simulink model "PurePursuit"  (R2020b)
settings: Solver=VariableStepAuto  StartTime=0  StopTime=10  RelTol=1e-3
undefined symbols (not defined in the file or in its folder): map, parking_space, start_pos
libraries: Solver_SF x1
settings Model: Creator=ASCL-321  LastModifiedBy=ASCL-321

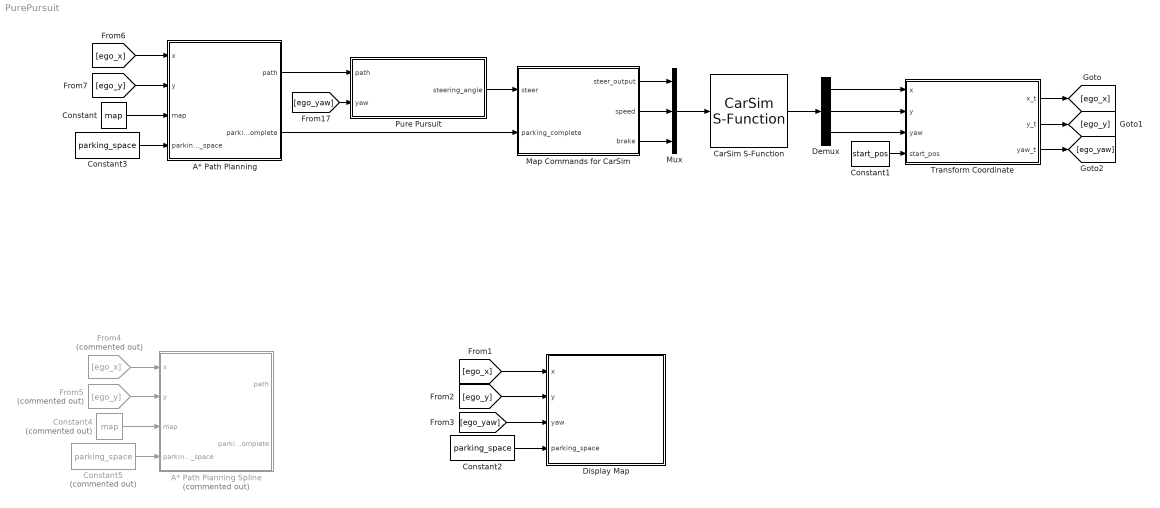
== system PurePursuit ==
  A* Path Planning : MATLAB Function  TreatAsAtomicUnit=on  SystemSampleTime=0.1
  A* Path Planning Spline : MATLAB Function  Commented=on  TreatAsAtomicUnit=on  SystemSampleTime=0.1
  CarSim S-Function : Solver_SF/CarSim S-Function  Priority=1  SIMFILE=simfile.sim  Run_RTs=off  vs_state_ind=Run  StopMode_ind=Vehicle Model
  Constant : Constant  Value=map
  Constant1 : Constant  Value=start_pos
  Constant2 : Constant  Value=parking_space
  Constant3 : Constant  Value=parking_space
  Constant4 : Constant  Commented=on  Value=map
  Constant5 : Constant  Commented=on  Value=parking_space
  Demux : Demux  Outputs=3
  Display Map : MATLAB Function  TreatAsAtomicUnit=on  SystemSampleTime=0.1
  From4 : From  Commented=on  GotoTag=ego_x
  From5 : From  Commented=on  GotoTag=ego_y
  Map Commands for CarSim : MATLAB Function  TreatAsAtomicUnit=on  SystemSampleTime=0.1
  Mux : Mux  Inputs=3
  Pure Pursuit : MATLAB Function  TreatAsAtomicUnit=on  SystemSampleTime=0.1
  Transform Coordinate : MATLAB Function  TreatAsAtomicUnit=on  SystemSampleTime=0.1
  wires:
  Map Commands for CarSim/1(steer_output) -> Mux/1
  Map Commands for CarSim/2(speed) -> Mux/2
  Mux/1 -> CarSim S-Function/1
  A* Path Planning/1(path) -> Pure Pursuit/1(path)
  CarSim S-Function/1 -> Demux/1
  Demux/1 -> Transform Coordinate/1(x)
  Demux/2 -> Transform Coordinate/2(y)
  [ego_yaw] -> Pure Pursuit/2(yaw)
  [ego_x] -> Display Map/1(x)
  [ego_y] -> Display Map/2(y)
  Demux/3 -> Transform Coordinate/3(yaw)
  [ego_yaw] -> Display Map/3(yaw)
  Transform Coordinate/3(yaw_t) -> [ego_yaw]
  Transform Coordinate/1(x_t) -> [ego_x]
  Transform Coordinate/2(y_t) -> [ego_y]
  Map Commands for CarSim/3(brake) -> Mux/3
  A* Path Planning/2(parking_complete) -> Map Commands for CarSim/2(parking_complete)
  Constant1/1 -> Transform Coordinate/4(start_pos)
  Constant2/1 -> Display Map/4(parking_space)
  Pure Pursuit/1(steering_angle) -> Map Commands for CarSim/1(steer)
  Constant/1 -> A* Path Planning/3(map)
  [ego_x] -> A* Path Planning/1(x)
  Constant3/1 -> A* Path Planning/4(parking_space)
  [ego_y] -> A* Path Planning/2(y)
  Constant5/1 -> A* Path Planning Spline/4(parking_space)
  From4/1 -> A* Path Planning Spline/1(x)
  From5/1 -> A* Path Planning Spline/2(y)
  Constant4/1 -> A* Path Planning Spline/3(map)

== matlab function PurePursuit/Display Map ==
  data: x input; y input; yaw input; parking_space input
function DisplayMap(x, y, yaw, parking_space)
%% Map parameters
lanethickness = 0.2;
parkingwidth = 2.3;
parkinglength = 5;

parkinglane_h = [lanethickness/2, lanethickness/2 + parkinglength];
parkinglane_v = [lanethickness/2, lanethickness/2];

goalx = (parkinglength + lanethickness)/2;
goaly = parkingwidth*(parking_space - 1) + (parkingwidth + lanethickness)/2;

linewidth = 3;

%% Plot map

figure(2);
plot([lanethickness/2, lanethickness/2], [lanethickness/2, lanethickness/2 + parkingwidth*5], 'k', 'LineWidth', linewidth); % Plot lanes
xlim([0,15.1])
ylim([0,11.7])
hold on
for i = 0: 5    
    plot(parkinglane_h, parkinglane_v + parkingwidth*i,'k', 'LineWidth', linewidth) % Plot lanes
    if parking_space ~= i && i ~= 0
        plotTarget((parkinglength + lanethickness)/2, parkingwidth*(i-1) + (parkingwidth + lanethickness)/2) % Plot parked vehicles
    end
end

plotEgo(x,y,yaw)
plot(goalx, goaly, 'gx')
hold off


function plotEgo(x,y,yaw)
ego_length = 2.6;
ego_width = 1.8;

h=sqrt((ego_length/2)^2+(ego_width/2)^2);
theta = atan(ego_width/ego_length);
psi=theta-yaw;
x1=x-h*cos(psi);
y1=y+h*sin(psi);
x2=x1+ego_length*cos(yaw);
y2=y1+ego_length*sin(yaw);
x3=2*x-x2;
y3=2*y-y2;
x4=x3+ego_length*cos(yaw);
y4=y3+ego_length*sin(yaw);

plot([x1 x2],[y1 y2], 'b')
plot([x3 x4],[y3 y4], 'b')
plot([x1 x3],[y1 y3], 'b')
plot([x2 x4],[y2 y4], 'b')

function plotTarget(target_x,target_y)
targetwidth = 1.8;
targetlength = 2.6;
plot([target_x - targetlength/2, target_x + targetlength/2], [target_y - targetwidth/2, target_y - targetwidth/2], 'r')
plot([target_x - targetlength/2, target_x + targetlength/2], [target_y + targetwidth/2, target_y + targetwidth/2], 'r')
plot([target_x - targetlength/2, target_x - targetlength/2], [target_y - targetwidth/2, target_y + targetwidth/2], 'r')
plot([target_x + targetlength/2, target_x + targetlength/2], [target_y - targetwidth/2, target_y + targetwidth/2], 'r')

== matlab function PurePursuit/Transform Coordinate ==
  data: x_t output; y_t output; x input; y input; yaw input; yaw_t output; start_pos input
function [x_t, y_t, yaw_t] = TransformCoordinate(x, y, yaw, start_pos)
theta = pi/2;

x_t = x*cos(theta) - y*sin(theta) + start_pos(1);
y_t = x*sin(theta) + y*cos(theta) + start_pos(2);

if -180 < yaw && yaw < 90
    yaw_t = (yaw + 90)*pi/180;
else
    yaw_t = (yaw - 270)*pi/180;
end

== matlab function PurePursuit/Map Commands for CarSim ==
  data: steer input; steer_output output; speed output; brake output; parking_complete input
function [steer_output, speed, brake] = fcn(steer, parking_complete)
brake = 0;
steer_output= -steer * 180/pi*15;

if parking_complete
    speed = 0;
    brake = 3;
else
    speed=5;
end

== matlab function PurePursuit/A* Path Planning ==
  data: x input; path output; y input; map input; parking_complete output; parking_space input
function [path, parking_complete] = fcn(x, y, map, parking_space)
res=100;
lanethickness = 0.2;
parkingwidth = 2.3;
parkinglength = 5;

goalx = res*(parkinglength + lanethickness)/2;
goaly = res*(parkingwidth*(parking_space-1) + (parkingwidth + lanethickness)/2);

ego_x = round(res*x);
ego_y = round(res*y);

x_path = zeros(556,1);
y_path = zeros(556,1);
x_path_global = zeros(556,1);
y_path_global = zeros(556,1);

parking_complete = 0;
if (goalx-ego_x)^2 + (goaly-ego_y)^2 < 2000
    parking_complete = 1;
end

for n = 1:556 % 2.78 m/s * 1s *2 preview time
    min = 1000000;
    min_i = ego_x;
    min_j = ego_y;
    for i = ego_x - 1: ego_x + 1
        for j = ego_y - 1: ego_y + 1
            buffer = sqrt((goalx - i)^2 + (goaly - j)^2);
            buffer = buffer + map(j,i)*buffer;
            if (buffer < min)
                min = buffer;
                min_i = i;
                min_j = j;
            end
        end
    end
    ego_x = min_i;
    ego_y = min_j;
    x_path(n) = (ego_x - round(res*x));
    y_path(n) = (ego_y - round(res*y));
    x_path_global(n) = ego_x;
    y_path_global(n) = ego_y;
end

hold on
plot(x_path_global/res,y_path_global/res, 'k')
hold off

path = [x_path, y_path];

== matlab function PurePursuit/A* Path Planning Spline ==
  data: x input; path output [..600]; y input; map input; parking_complete output; parking_space input
function [path, parking_complete] = fcn(x, y, map, parking_space)
res=100;
lanethickness = 0.2;
parkingwidth = 2.3;
parkinglength = 5;

goalx = res*(parkinglength + lanethickness)/2;
goaly = res*(parkingwidth*(parking_space-1) + (parkingwidth + lanethickness)/2);

ego_x = round(res*x);
ego_y = round(res*y);

x_path = zeros(556,1);
y_path = zeros(556,1);
x_path_global = [ ];
y_path_global = [ ];

parking_complete = 0;
if (goalx-ego_x)^2 + (goaly-ego_y)^2 < 2000
    parking_complete = 1;
end

for n = 1:556 % 2.78 m/s * 1s *2 preview time
    min = 1000000;
    min_i = ego_x;
    min_j = ego_y;
    if ego_x - 1 > 0 && ego_x + 1 < 1510
        for i = ego_x - 1: ego_x + 1
            for j = ego_y - 1: ego_y + 1
                buffer = sqrt((goalx - i)^2 + (goaly - j)^2);
                buffer = buffer + map(j,i)*buffer;
                if (buffer < min)
                    min = buffer;
                    min_i = i;
                    min_j = j;
                end
            end
        end
    end
    
    if min_i == ego_x && min_j == ego_y
        continue
    end

    ego_x = min_i;
    ego_y = min_j;
    x_path(n) = (ego_x - round(x*res));
    y_path(n) = (ego_y - round(y*res));
    x_path_global = [x_path_global ego_x];
    y_path_global = [y_path_global ego_y];
        
end

temp = length(x_path_global);
yy = spline([x_path_global(temp) x_path_global(round(temp/2)) x_path_global(1)], [y_path_global(temp) y_path_global(round(temp/2)) y_path_global(1)], x_path_global);

temp = length(x_path);

hold on
plot(x_path_global/res,y_path_global/res, 'k')
plot(x_path_global/res, yy/res)
hold off

path = [x_path, y_path];

== matlab function PurePursuit/Pure Pursuit ==
  data: path input; steering_angle output; yaw input
function steering_angle  = fcn(path, yaw)
res=100;
ld = 4*0.5*res;   % Look ahead distance as a hyperparameter, 0.5s preview time
L = 2.35*res; % wheel base
rear_center = [- L/2*cos(yaw), - L/2*sin(yaw)]; % Rear wheels' center

min = 1000000;
min_n = 1;
for n = 1:556
    buffer = sqrt((rear_center(1)-path(n,1))^2 + (rear_center(2)-path(n,2))^2);
    if (abs(buffer - ld) < min)
        min = abs(buffer - ld);
        min_n = n;
    end
end

p_x = path(min_n,1);
p_y = path(min_n,2);

alpha = atan(p_y/p_x) - yaw;
steering_angle = atan(2*L*sin(alpha)/ld);
